simulink model "proc_control_lite"  (R2024b)
settings: Solver=FixedStepAuto  StartTime=0.0  StopTime=inf  RelTol=1e-3
InitFcn:
  | InitProcControl;
StartFcn:
  | LoadParams;
model workspace (MAT data in the model file):
  SL_ROS_VariableLengthArrays_MaxSizes : object (value not decoded)
values from neighbouring files (symbols this model uses):
  A = T200Spec16V{:,3}    [InitProcControl.m]
  N = T200Spec16V{:,6}    [InitProcControl.m]
  PWM = T200Spec16V{:,1}    [InitProcControl.m]
undefined symbols (not defined in the file or in its folder): config, current_gains, DiscIntNeverNeededParam, is_mpc_alive, is_trajectory_done, motor1, motor2, motor3, motor4, motor5, motor6, motor7, motor8, MPC, mpc_mode, mpc_status, orientation, physics, pose, position, simulation, simulink, target_reached, thrusters_status, thrusters_status_SL_Info, twist
libraries: ros2lib x64, dspstat3 x24, aerolibutil x15, dspfdesign x7, simulink x5, mpclib x3, matrix_library x3, robotcorelib x2, sharedtransform x1, sharedTrackingLibrary x1
(part 2 of 3)

== system proc_control_lite/Subsystem Trajectory/ProcPlanner Trajectory ==
  isNew : Inport
  trajMsg : Inport  Port=2
  output : Inport  Port=3
  reset : Inport  Port=4
  rosParam : Inport  Port=5
  Action Port : ActionPort  ActionPortLabel=case [ 10 ]:
  Bus Creator : BusCreator  Inputs=4
  Bus Selector : BusSelector  OutputSignals=WorldPosition,qS2W,Body Velocity,Angular Rate  OutputAsBus=on
  Detect Rise Positive : simulink/Logic and Bit Operations/Detect Rise Positive  vinit=0  OutDataTypeStr=boolean
  MATLAB System : MATLABSystem  System=ProcPlannerManager  mpcConst=MPC  SimulateUsing=Code generation
      mask Type: ProcPlannerManager
      mask Display:
      | disp('ProcPlannerManager');
      | port_label('input',1,'isNew');
      | port_label('input',2,'trajMsg');
      | port_label('input',3,'reset');
      | port_label('input',4,'mesuredPose');
      | port_label('input',5,'mpcParams');
      | port_label('output',1,'currentPose');
      | port_label('output',2,'isReached');
      | port_label('output',3,'isTrajDone');
      | port_label('output',4,'initWpt');
  Refrence : Outport
  wires:
  isNew/1 -> Detect Rise Positive/1
  Detect Rise Positive/1 -> MATLAB System/1
  trajMsg/1 -> MATLAB System/2
  reset/1 -> MATLAB System/3
  output/1 -> Bus Selector/1
  Bus Selector/1 -> MATLAB System/4
  rosParam/1 -> MATLAB System/5
  MATLAB System/4 -> Bus Creator/4  "target"
  MATLAB System/3 -> Bus Creator/3  "isTrajDone"
  MATLAB System/2 -> Bus Creator/2  "isReached"
  MATLAB System/1 -> Bus Creator/1  "Reference"
  Bus Creator/1 -> Refrence/1

== system proc_control_lite/Subsystem Trajectory/Send Current Target ==
  pose : Inport
  Blank Message : ros2lib/Blank Message  messageClass=Message  entityType=geometry_msgs/Pose  messageType=geometry_msgs/Pose  SampleTime=inf
  Bus Assignment : BusAssignment  AssignedSignals=position.x,position.y,position.z,orientation.w,orientation.x,orientation.y,orientation.z
  Demux : Demux  Outputs=7
  Publish : ros2lib/Publish  topicSource=Specify your own  topic=/proc_control/current_target  messageType=geometry_msgs/Pose  QOSHistory=Keep last  QOSDepth=1  QOSReliability=Reliable  QOSDurability=Volatile  QOSDeadline=Inf  QOSLifespan=5  QOSLiveliness=Automatic  QOSLeaseDuration=5  QOSAvoidROSNamespaceConventions=off
  Zero-Order Hold : ZeroOrderHold
  wires:
  Blank Message/1 -> Bus Assignment/1
  pose/1 -> Demux/1
  Demux/1 -> Bus Assignment/2
  Demux/2 -> Bus Assignment/3
  Demux/3 -> Bus Assignment/4
  Demux/4 -> Bus Assignment/5
  Demux/5 -> Bus Assignment/6
  Demux/6 -> Bus Assignment/7
  Demux/7 -> Bus Assignment/8
  Bus Assignment/1 -> Zero-Order Hold/1
  Zero-Order Hold/1 -> Publish/1

== system proc_control_lite/Subsystem Trajectory/SpaceNav ==
  y : Inport
  Action Port : ActionPort  ActionPortLabel=case [ 19 20 21 ]:
  Bus Creator : BusCreator  Inputs=4
  Constant : Constant  Value=[0 0 0 1 0 0 0]
  Constant1 : Constant  Value=MPC.p
  Constant2 : Constant  Value=false  VectorParams1D=off
  Constant3 : Constant  Value=false  VectorParams1D=off
  MATLAB Function : MATLAB Function  TreatAsAtomicUnit=on
  Mux : Mux  Inputs=2
  Selector : Selector  InputPortWidth=13  IndexOptions=Index vector (dialog)  Indices=[1:7]  OutputSizes=1
  Transpose : Math  Operator=transpose  OutputSignalType=real
  Out1 : Outport
  wires:
  Constant/1 -> Mux/1
  y/1 -> Mux/2
  Mux/1 -> Transpose/1
  Transpose/1 -> Selector/1, MATLAB Function/1(matrix)
  Constant1/1 -> MATLAB Function/2(p)
  MATLAB Function/1(y) -> Bus Creator/1  "Reference"
  Selector/1 -> Bus Creator/4  "target"
  Constant3/1 -> Bus Creator/3  "isTrajDone"
  Constant2/1 -> Bus Creator/2  "isReached"
  Bus Creator/1 -> Out1/1

== system proc_control_lite/Subsystem Trajectory/Subsystem ==
  Bus Selector : BusSelector  OutputSignals=linear.x,linear.y,linear.z  OutputAsBus=on
  Bus Selector1 : BusSelector  OutputSignals=angular.x,angular.y,angular.z  OutputAsBus=on
  Bus to Vector : BusToVector
  Bus to Vector1 : BusToVector
  Gain : Gain  Gain=-1
  Mux : Mux  Inputs=2
  Scope : Scope
  Subscribe : ros2lib/Subscribe  topicSource=Specify your own  topic=/spacenav/twist  messageType=geometry_msgs/Twist  sampleTime=1/25  QOSHistory=Keep last  QOSDepth=1  QOSReliability=Reliable  QOSDurability=Volatile  QOSDeadline=Inf  QOSLifespan=5  QOSLiveliness=Automatic  QOSLeaseDuration=5  QOSAvoidROSNamespaceConventions=off
  Terminator : Terminator
  y : Outport
  wires:
  Subscribe/1 -> Terminator/1
  Subscribe/2 -> Bus Selector1/1, Bus Selector/1
  Bus Selector/1 -> Bus to Vector/1
  Bus Selector1/1 -> Bus to Vector1/1
  Bus to Vector1/1 -> Gain/1
  Bus to Vector/1 -> Mux/1
  Gain/1 -> Mux/2
  Mux/1 -> Scope/1, y/1

== system proc_control_lite/Subsystem Trajectory/Subsystem1 ==
  Subscribe : ros2lib/Subscribe  topicSource=Specify your own  topic=/proc_planner/send_trajectory_list  messageType=trajectory_msgs/MultiDOFJointTrajectoryPoint  sampleTime=1  QOSHistory=Keep last  QOSDepth=1  QOSReliability=Reliable  QOSDurability=Volatile  QOSDeadline=Inf  QOSLifespan=inf  QOSLiveliness=Automatic  QOSLeaseDuration=Inf  QOSAvoidROSNamespaceConventions=off
  isNew : Outport
  trajMsg : Outport  Port=2
  wires:
  Subscribe/1 -> isNew/1
  Subscribe/2 -> trajMsg/1

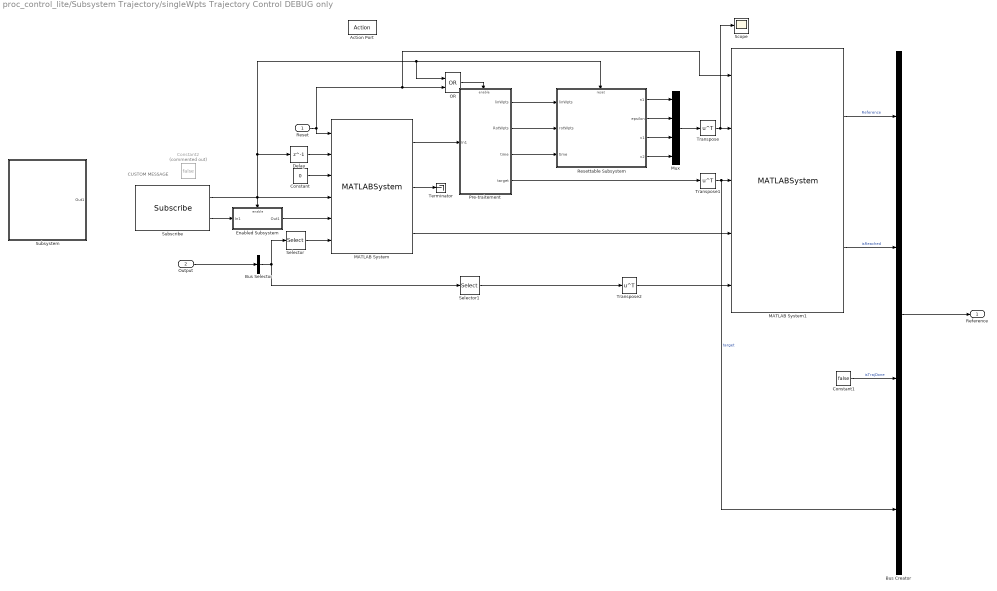
== system proc_control_lite/Subsystem Trajectory/singleWpts Trajectory Control DEBUG only ==
  note: CUSTOM MESSAGE
  Reset : Inport
  Output : Inport  Port=2
  Action Port : ActionPort  InitializeStates=reset  ActionPortLabel=case [ 11 30 31 40 41 ]:
  Bus Creator : BusCreator  Inputs=4
  Bus Selector : BusSelector  OutputSignals=WorldPosition,qS2W,Body Velocity,Angular Rate  OutputAsBus=on
  Constant : Constant  Value=0
  Constant1 : Constant  Value=false
  Constant2 : Constant  Commented=on  Value=false
  Delay : Delay  DelayLength=1
  Enabled Subsystem : Subsystem  TreatAsAtomicUnit=on
  MATLAB System : MATLABSystem  System=AddPose  buffSize=2  elementSize=9  SimulateUsing=Code generation
      mask Type: AddPose
      mask Display:
      | disp('AddPose');
      | port_label('input',1,'reset');
      | port_label('input',2,'compute');
      | port_label('input',3,'clearBuffer');
      | port_label('input',4,'isNew');
      | port_label('input',5,'waypoint');
      | port_label('input',6,'xk');
      | port_label('output',1,'waypoints');
      | port_label('output',2,'count');
      | port_label('output',3,'initCond');
  MATLAB System1 : MATLABSystem  System=TrajectoryManager  SampleTime=MPC.Ts  OffsetTime=0  prediction=MPC.p  bufferSize=6001  linearConvergence=.25  quaternionConvergence=.22  TargetThreshold=2  SimulateUsing=Code generation
      mask Type: TrajectoryManager
      mask Display:
      | disp('TrajectoryManager');
      | port_label('input',1,'reset');
      | port_label('input',2,'poses');
      | port_label('input',3,'target');
      | port_label('input',4,'x0');
      | port_label('input',5,'mesuredPose');
      | port_label('output',1,'currentPose');
      | port_label('output',2,'isReached');
  Mux : Mux
  OR : Logic  Operator=OR  IconShape=distinctive  AllPortsSameDT=off  OutDataTypeStr=boolean
  Pre-traitement : Subsystem  TreatAsAtomicUnit=on
  Resettable Subsystem : Subsystem  TreatAsAtomicUnit=on
  Scope : Scope
  Selector : Selector  InputPortWidth=13  IndexOptions=Index vector (dialog)  Indices=[1:7]  OutputSizes=1
  Selector1 : Selector  InputPortWidth=13  IndexOptions=Index vector (dialog)  Indices=[1:13]  OutputSizes=1
  Subscribe : ros2lib/Subscribe  topicSource=Specify your own  topic=/proc_control/add_pose  messageType=sonia_common_ros2/Pose  sampleTime=-1  QOSHistory=Keep last  QOSDepth=1  QOSReliability=Reliable  QOSDurability=Volatile  QOSDeadline=Inf  QOSLifespan=inf  QOSLiveliness=Automatic  QOSLeaseDuration=inf  QOSAvoidROSNamespaceConventions=off
  Subsystem : Subsystem
  Terminator : Terminator
  Transpose : Math  Operator=transpose
  Transpose1 : Math  Operator=transpose
  Transpose2 : Math  Operator=transpose
  Reference : Outport
  wires:
  Reset/1 -> MATLAB System1/1, OR/2, MATLAB System/1
  Subscribe/1 -> Resettable Subsystem/Reset, OR/1, Delay/1, Enabled Subsystem/Enable, MATLAB System/4
  Enabled Subsystem/1(Out1) -> MATLAB System/5
  Constant/1 -> MATLAB System/3
  Delay/1 -> MATLAB System/2
  MATLAB System/2 -> Terminator/1
  Output/1 -> Bus Selector/1
  Bus Selector/1 -> Selector/1, Selector1/1
  Selector/1 -> MATLAB System/6
  MATLAB System/1 -> Pre-traitement/1(In1)
  OR/1 -> Pre-traitement/Enable
  Pre-traitement/1(linWpts) -> Resettable Subsystem/1(linWpts)
  Pre-traitement/2(RotWpts) -> Resettable Subsystem/2(rotWpts)
  Pre-traitement/3(time) -> Resettable Subsystem/3(time)
  Resettable Subsystem/1(n1) -> Mux/1
  Resettable Subsystem/2(epsilon) -> Mux/2
  Resettable Subsystem/3(v1) -> Mux/3
  Resettable Subsystem/4(v2) -> Mux/4
  Mux/1 -> Transpose/1
  Transpose/1 -> Scope/1, MATLAB System1/2
  Pre-traitement/4(target) -> Transpose1/1
  Transpose1/1 -> Bus Creator/4, MATLAB System1/3  "target"
  MATLAB System/3 -> MATLAB System1/4
  Transpose2/1 -> MATLAB System1/5
  Selector1/1 -> Transpose2/1
  MATLAB System1/1 -> Bus Creator/1  "Reference"
  MATLAB System1/2 -> Bus Creator/2  "isReached"
  Constant1/1 -> Bus Creator/3  "isTrajDone"
  Bus Creator/1 -> Reference/1
  Subscribe/2 -> Enabled Subsystem/1(In1)

== system proc_control_lite/Enabled Subsystem/Send auv states/bus2mux ==
  Input : Inport
  Bus Selector : BusSelector  OutputSignals=WorldPosition,qS2W,Body Velocity,Angular Rate
  Mux : Mux
  states : Outport
  wires:
  Bus Selector/1 -> Mux/1  "<WorldPosition>"
  Input/1 -> Bus Selector/1
  Bus Selector/2 -> Mux/2  "<qS2W>"
  Mux/1 -> states/1
  Bus Selector/3 -> Mux/3  "<Body Velocity>"
  Bus Selector/4 -> Mux/4  "<Angular Rate>"

== system proc_control_lite/Ros Command/Get_ROS_param/MPC Parameters ==
  Bus Creator : BusCreator  Inputs=2  OutDataTypeStr=Bus: mpcParams
  MPC Gains : Subsystem
  targetReached Params : Subsystem
  mpcParams : Outport
  wires:
  MPC Gains/1(gains) -> Bus Creator/1
  targetReached Params/1(targetReached) -> Bus Creator/2
  Bus Creator/1 -> mpcParams/1  "mpcParams"

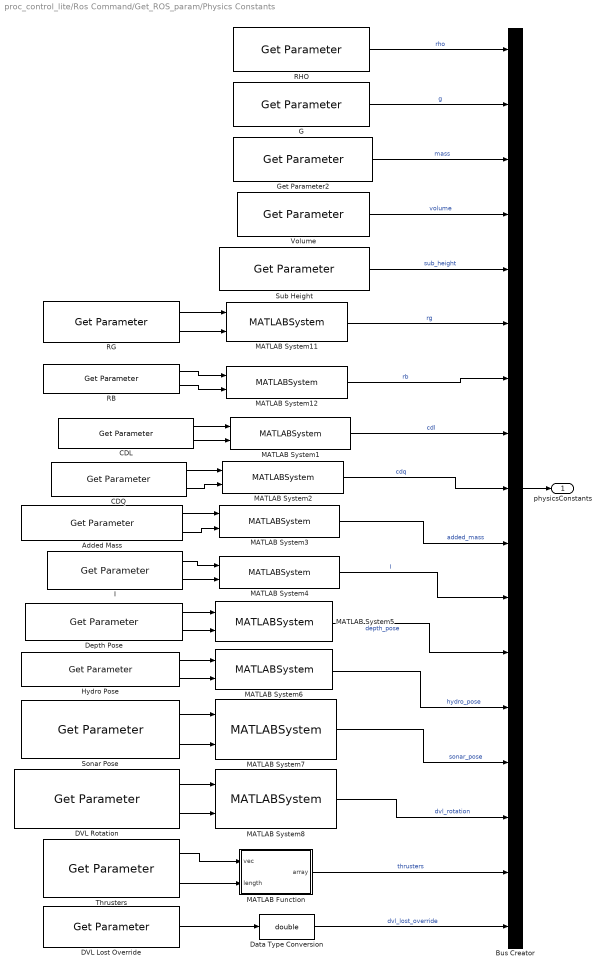
== system proc_control_lite/Ros Command/Get_ROS_param/Physics Constants ==
  Added Mass : ros2lib/Get Parameter  ParameterName=proc_control.physics.added_mass  ParameterType=double[]  ParameterMaxArrayLength=64  ParameterInitialValue=int8([0,0,0,0,0,0])  SampleTime=-1  ModelName=proc_control_lite  BlockId=ParamGet_proc_control_lite_180
  Bus Creator : BusCreator  Inputs=17  OutDataTypeStr=Bus: physicsConstants  NonVirtualBus=on
  CDL : ros2lib/Get Parameter  ParameterName=proc_control.physics.cdl  ParameterType=double[]  ParameterMaxArrayLength=64  ParameterInitialValue=int8([0,0,0,0,0,0])  SampleTime=-1  ModelName=proc_control_lite  BlockId=ParamGet_proc_control_lite_175
  CDQ : ros2lib/Get Parameter  ParameterName=proc_control.physics.cdq  ParameterType=double[]  ParameterMaxArrayLength=64  ParameterInitialValue=int8([0,0,0,0,0,0])  SampleTime=-1  ModelName=proc_control_lite  BlockId=ParamGet_proc_control_lite_177
  DVL Lost Override : ros2lib/Get Parameter  ParameterName=proc_control.physics.dvl_lost_override  ParameterType=boolean  ParameterMaxArrayLength=16  ParameterInitialValue=true  SampleTime=-1  ModelName=proc_control_lite  BlockId=ParamGet_proc_control_lite_196
  DVL Rotation : ros2lib/Get Parameter  ParameterName=proc_control.physics.dvl_rotation  ParameterType=double[]  ParameterMaxArrayLength=64  ParameterInitialValue=int8([0,0,0])  SampleTime=-1  ModelName=proc_control_lite  BlockId=ParamGet_proc_control_lite_192
  Data Type Conversion : DataTypeConversion  OutDataTypeStr=double  SaturateOnIntegerOverflow=off  RndMeth=Floor
  Depth Pose : ros2lib/Get Parameter  ParameterName=proc_control.physics.depth_pose  ParameterType=double[]  ParameterMaxArrayLength=64  ParameterInitialValue=int8([0,0,0])  SampleTime=-1  ModelName=proc_control_lite  BlockId=ParamGet_proc_control_lite_184
  G : ros2lib/Get Parameter  ParameterName=proc_control.physics.g  ParameterType=double  ParameterMaxArrayLength=16  ParameterInitialValue=physics.g  SampleTime=-1  ModelName=proc_control_lite  BlockId=ParamGet_proc_control_lite_167
  Get Parameter2 : ros2lib/Get Parameter  ParameterName=proc_control.physics.mass  ParameterType=double  ParameterMaxArrayLength=16  ParameterInitialValue=physics.mass  SampleTime=-1  ModelName=proc_control_lite  BlockId=ParamGet_proc_control_lite_168
  Hydro Pose : ros2lib/Get Parameter  ParameterName=proc_control.physics.hydro_pose  ParameterType=double[]  ParameterMaxArrayLength=64  ParameterInitialValue=int8([0,0,0])  SampleTime=-1  ModelName=proc_control_lite  BlockId=ParamGet_proc_control_lite_186
  I : ros2lib/Get Parameter  ParameterName=proc_control.physics.I  ParameterType=double[]  ParameterMaxArrayLength=128  ParameterInitialValue=int8([0,0,0,0,0,0,0,0,0])  SampleTime=-1  ModelName=proc_control_lite  BlockId=ParamGet_proc_control_lite_182
  MATLAB Function : MATLAB Function  TreatAsAtomicUnit=on
  MATLAB System1 : MATLABSystem  System=Vector2DoubleArray  arraySize=[1, 6]  constantName='Linear drag constant'  SimulateUsing=Code generation
      mask Type: Vector2DoubleArray
      mask Display:
      | disp('Vector2DoubleArray');
      | port_label('input',1,'vector');
      | port_label('input',2,'length');
      | port_label('output',1,'array');
  MATLAB System11 : MATLABSystem  System=Vector2DoubleArray  arraySize=[1 3]  constantName='Center of Mass'  SimulateUsing=Code generation
      mask Type: Vector2DoubleArray
      mask Display:
      | disp('Vector2DoubleArray');
      | port_label('input',1,'vector');
      | port_label('input',2,'length');
      | port_label('output',1,'array');
  MATLAB System12 : MATLABSystem  System=Vector2DoubleArray  arraySize=[1, 3]  constantName='Center of Buoyancy'  SimulateUsing=Code generation
      mask Type: Vector2DoubleArray
      mask Display:
      | disp('Vector2DoubleArray');
      | port_label('input',1,'vector');
      | port_label('input',2,'length');
      | port_label('output',1,'array');
  MATLAB System2 : MATLABSystem  System=Vector2DoubleArray  arraySize=[1, 6]  constantName='Quadratic drag constant'  SimulateUsing=Code generation
      mask Type: Vector2DoubleArray
      mask Display:
      | disp('Vector2DoubleArray');
      | port_label('input',1,'vector');
      | port_label('input',2,'length');
      | port_label('output',1,'array');
  MATLAB System3 : MATLABSystem  System=Vector2DoubleArray  arraySize=[1, 6]  constantName='Added Mass'  SimulateUsing=Code generation
      mask Type: Vector2DoubleArray
      mask Display:
      | disp('Vector2DoubleArray');
      | port_label('input',1,'vector');
      | port_label('input',2,'length');
      | port_label('output',1,'array');
  MATLAB System4 : MATLABSystem  System=Vector2DoubleArray  arraySize=[1,9]  constantName='Inertia Tensor'  SimulateUsing=Code generation
      mask Type: Vector2DoubleArray
      mask Display:
      | disp('Vector2DoubleArray');
      | port_label('input',1,'vector');
      | port_label('input',2,'length');
      | port_label('output',1,'array');
  MATLAB System5 : MATLABSystem  System=Vector2DoubleArray  arraySize=[1 3]  constantName='Depth Pose'  SimulateUsing=Code generation
      mask Type: Vector2DoubleArray
      mask Display:
      | disp('Vector2DoubleArray');
      | port_label('input',1,'vector');
      | port_label('input',2,'length');
      | port_label('output',1,'array');
  MATLAB System6 : MATLABSystem  System=Vector2DoubleArray  arraySize=[1, 3]  constantName='Hydro Pose'  SimulateUsing=Code generation
      mask Type: Vector2DoubleArray
      mask Display:
      | disp('Vector2DoubleArray');
      | port_label('input',1,'vector');
      | port_label('input',2,'length');
      | port_label('output',1,'array');
  MATLAB System7 : MATLABSystem  System=Vector2DoubleArray  arraySize=[1, 3]  constantName='Sonar Pose'  SimulateUsing=Code generation
      mask Type: Vector2DoubleArray
      mask Display:
      | disp('Vector2DoubleArray');
      | port_label('input',1,'vector');
      | port_label('input',2,'length');
      | port_label('output',1,'array');
  MATLAB System8 : MATLABSystem  System=Vector2DoubleArray  arraySize=[1, 3]  constantName='DVL Rotation'  SimulateUsing=Code generation
      mask Type: Vector2DoubleArray
      mask Display:
      | disp('Vector2DoubleArray');
      | port_label('input',1,'vector');
      | port_label('input',2,'length');
      | port_label('output',1,'array');
  RB : ros2lib/Get Parameter  ParameterName=proc_control.physics.rb  ParameterType=double[]  ParameterMaxArrayLength=64  ParameterInitialValue=int8([0,0,0])  SampleTime=-1  ModelName=proc_control_lite  BlockId=ParamGet_proc_control_lite_173
  RG : ros2lib/Get Parameter  ParameterName=proc_control.physics.rg  ParameterType=double[]  ParameterMaxArrayLength=64  ParameterInitialValue=double([0,0,0])  SampleTime=-1  ModelName=proc_control_lite  BlockId=ParamGet_proc_control_lite_171
  RHO : ros2lib/Get Parameter  ParameterName=proc_control.physics.rho  ParameterType=double  ParameterMaxArrayLength=16  ParameterInitialValue=physics.rho  SampleTime=-1  ModelName=proc_control_lite  BlockId=ParamGet_proc_control_lite_166
  Sonar Pose : ros2lib/Get Parameter  ParameterName=proc_control.physics.sonar_pose  ParameterType=double[]  ParameterMaxArrayLength=64  ParameterInitialValue=int8([0,0,0])  SampleTime=-1  ModelName=proc_control_lite  BlockId=ParamGet_proc_control_lite_190
  Sub Height : ros2lib/Get Parameter  ParameterName=proc_control.physics.sub_height  ParameterType=double  ParameterMaxArrayLength=16  ParameterInitialValue=physics.height  SampleTime=-1  ModelName=proc_control_lite  BlockId=ParamGet_proc_control_lite_170
  Thrusters : ros2lib/Get Parameter  ParameterName=proc_control.physics.thrusters  ParameterType=double[]  ParameterMaxArrayLength=400  ParameterInitialValue=int8(zeros(1,48))  SampleTime=-1  ModelName=proc_control_lite  BlockId=ParamGet_proc_control_lite_194
  Volume : ros2lib/Get Parameter  ParameterName=proc_control.physics.volume  ParameterType=double  ParameterMaxArrayLength=16  ParameterInitialValue=physics.volume  SampleTime=-1  ModelName=proc_control_lite  BlockId=ParamGet_proc_control_lite_169
  physicsConstants : Outport
  wires:
  MATLAB System6/1 -> Bus Creator/13  "hydro_pose"
  CDL/2 -> MATLAB System1/2
  MATLAB System2/1 -> Bus Creator/9  "cdq"
  Thrusters/1 -> MATLAB Function/1(vec)
  RG/2 -> MATLAB System11/2
  CDQ/2 -> MATLAB System2/2
  Depth Pose/1 -> MATLAB System5/1
  MATLAB System8/1 -> Bus Creator/15  "dvl_rotation"
  CDL/1 -> MATLAB System1/1
  CDQ/1 -> MATLAB System2/1
  Added Mass/1 -> MATLAB System3/1
  Added Mass/2 -> MATLAB System3/2
  I/1 -> MATLAB System4/1
  I/2 -> MATLAB System4/2
  Depth Pose/2 -> MATLAB System5/2
  Hydro Pose/1 -> MATLAB System6/1
  Hydro Pose/2 -> MATLAB System6/2
  Sonar Pose/1 -> MATLAB System7/1
  Sonar Pose/2 -> MATLAB System7/2
  DVL Rotation/1 -> MATLAB System8/1
  DVL Rotation/2 -> MATLAB System8/2
  Thrusters/2 -> MATLAB Function/2(length)
  DVL Lost Override/1 -> Data Type Conversion/1
  RHO/1 -> Bus Creator/1  "rho"
  Sub Height/1 -> Bus Creator/5  "sub_height"
  G/1 -> Bus Creator/2  "g"
  Volume/1 -> Bus Creator/4  "volume"
  MATLAB System12/1 -> Bus Creator/7  "rb"
  MATLAB System1/1 -> Bus Creator/8  "cdl"
  MATLAB System3/1 -> Bus Creator/10  "added_mass"
  MATLAB System4/1 -> Bus Creator/11  "I"
  MATLAB System5/1 -> Bus Creator/12  "depth_pose"
  MATLAB System7/1 -> Bus Creator/14  "sonar_pose"
  MATLAB Function/1(array) -> Bus Creator/16  "thrusters"
  Data Type Conversion/1 -> Bus Creator/17  "dvl_lost_override"
  Bus Creator/1 -> physicsConstants/1
  Get Parameter2/1 -> Bus Creator/3  "mass"
  RG/1 -> MATLAB System11/1
  MATLAB System11/1 -> Bus Creator/6  "rg"
  RB/1 -> MATLAB System12/1
  RB/2 -> MATLAB System12/2

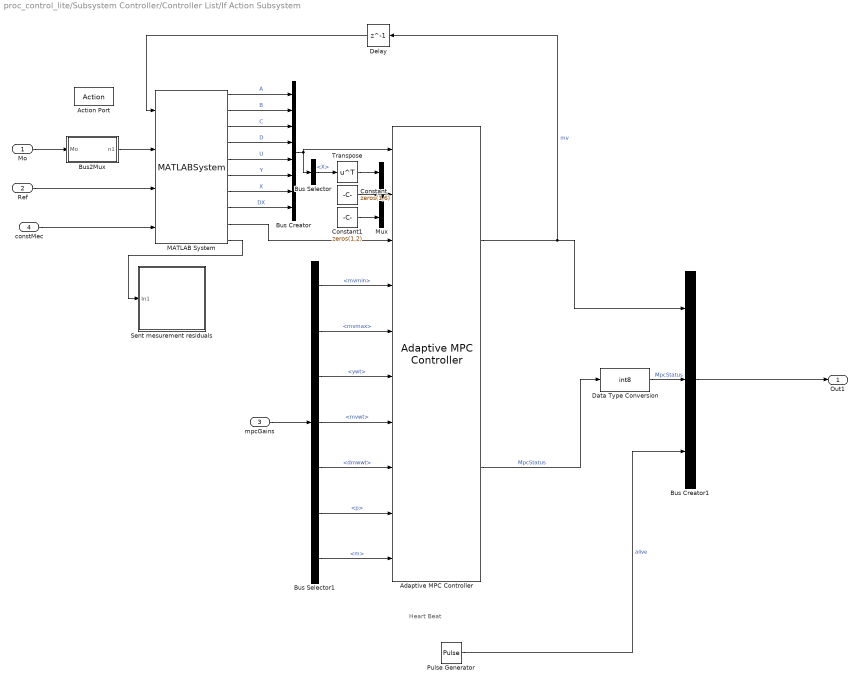
== system proc_control_lite/Subsystem Controller/Controller List/If Action Subsystem ==
  note: Heart Beat
  Mo : Inport
  Ref : Inport  Port=2
  mpcGains : Inport  Port=3
  constMec : Inport  Port=4
  Action Port : ActionPort  InitializeStates=reset  PropagateVarSize=During execution  ActionPortLabel=case [ 10 11 19 31 ]:
  Adaptive MPC Controller : mpclib/Adaptive MPC Controller  SCDEnableBlockLinearizationSpecification=on  mpcobj=Qmpcobj  enable_value=0  updateMPCinCallerWorkspace=on  md_inport=off  mv_inport=off  uref_inport=off  return_cost=off  return_mvseq=off  return_qpstatus=on  return_xseq=off  return_state=off  return_ovseq=off  state_inport=on  isltv_plant=off  umin_inport=on  umax_inport=on  ymin_inport=off  ymax_inport=off  cc_inport=off  ywt_inport=on  uwt_inport=on  duwt_inport=on  rhoeps_inport=off  pm_inport=on  MaximumP=10  HorizonChoice=VariableHorizon  BlockDataType=double  SampleTimeInherited=off  switch_inport=off
  Bus Creator : BusCreator  Inputs=8
  Bus Creator1 : BusCreator  Inputs=3
  Bus Selector : BusSelector  OutputSignals=X
  Bus Selector1 : BusSelector  OutputSignals=mvmin,mvmax,ywt,mvwt,dmwwt,p,m
  Bus2Mux : Subsystem
  Constant : Constant  Value=zeros(1,6)
  Constant1 : Constant  Value=zeros(1,2)
  Data Type Conversion : DataTypeConversion  OutDataTypeStr=int8  SaturateOnIntegerOverflow=off  RndMeth=Floor
  Delay : Delay  DelayLength=1  InitialCondition=zeros(MPC.nu,1)  SampleTime=MPC.Ts
  MATLAB System : MATLABSystem  System=TrimPlant  MPC=MPC  useDynamicsConst=on  SimulateUsing=Code generation
      mask Type: TrimPlant
      mask Display:
      | disp('TrimPlant');
      | port_label('input',1,'u');
      | port_label('input',2,'y');
      | port_label('input',3,'ref');
      | port_label('input',4,'constMec');
      | port_label('output',1,'A');
      | port_label('output',2,'B');
      | port_label('output',3,'C');
      | port_label('output',4,'D');
      | port_label('output',5,'U');
      | port_label('output',6,'Y');
      | port_label('output',7,'X');
      | port_label('output',8,'DX');
      | port_label('output',9,'ref');
      | port_label('output',10,'Z');
  Mux : Mux  Inputs=3
  Pulse Generator : DiscretePulseGenerator  SampleTime=MPC.Ts
  Sent mesurement residuals : Subsystem
  Transpose : Math  Operator=transpose
  Out1 : Outport
  wires:
  Mo/1 -> Bus2Mux/1(Mo)
  Bus2Mux/1(n1) -> MATLAB System/2
  Ref/1 -> MATLAB System/3
  constMec/1 -> MATLAB System/4
  MATLAB System/1 -> Bus Creator/1  "A"
  MATLAB System/2 -> Bus Creator/2  "B"
  MATLAB System/3 -> Bus Creator/3  "C"
  MATLAB System/4 -> Bus Creator/4  "D"
  MATLAB System/5 -> Bus Creator/5  "U"
  MATLAB System/6 -> Bus Creator/6  "Y"
  MATLAB System/7 -> Bus Creator/7  "X"
  MATLAB System/8 -> Bus Creator/8  "DX"
  Bus Creator/1 -> Bus Selector/1, Adaptive MPC Controller/1
  Constant/1 -> Mux/2
  Constant1/1 -> Mux/3
  Mux/1 -> Adaptive MPC Controller/2
  Bus Selector/1 -> Transpose/1  "<X>"
  Transpose/1 -> Mux/1
  MATLAB System/9 -> Adaptive MPC Controller/3
  mpcGains/1 -> Bus Selector1/1
  Bus Selector1/1 -> Adaptive MPC Controller/4  "<mvmin>"
  Bus Selector1/2 -> Adaptive MPC Controller/5  "<mvmax>"
  Bus Selector1/3 -> Adaptive MPC Controller/6  "<ywt>"
  Bus Selector1/4 -> Adaptive MPC Controller/7  "<mvwt>"
  Bus Selector1/5 -> Adaptive MPC Controller/8  "<dmwwt>"
  Bus Selector1/6 -> Adaptive MPC Controller/9  "<p>"
  Bus Selector1/7 -> Adaptive MPC Controller/10  "<m>"
  MATLAB System/10 -> Sent mesurement residuals/1(In1)
  Adaptive MPC Controller/1 -> Delay/1, Bus Creator1/1  "mv"
  Adaptive MPC Controller/2 -> Data Type Conversion/1  "MpcStatus"
  Pulse Generator/1 -> Bus Creator1/3  "alive"
  Delay/1 -> MATLAB System/1
  Bus Creator1/1 -> Out1/1
  Data Type Conversion/1 -> Bus Creator1/2  "MpcStatus"

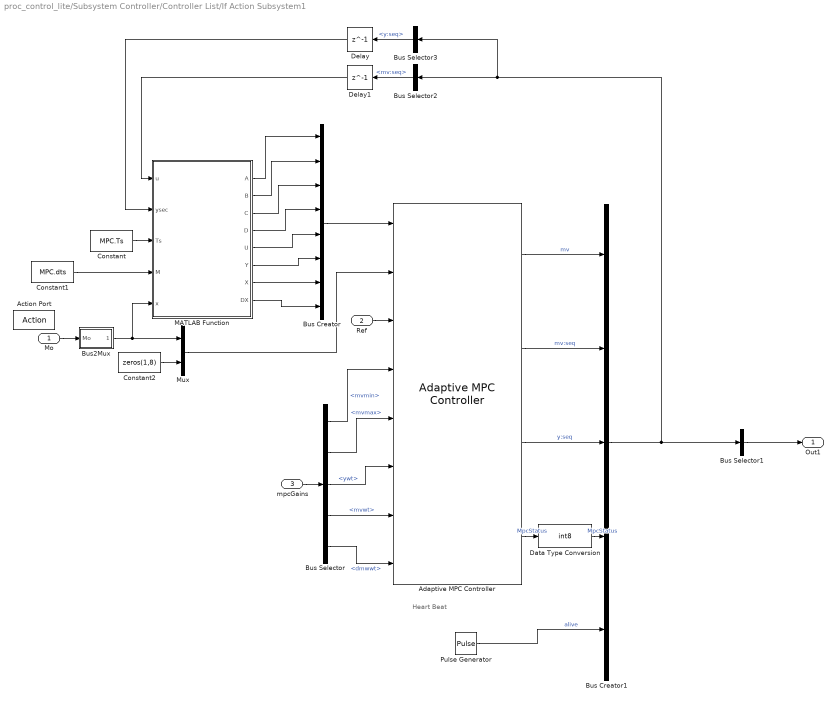
== system proc_control_lite/Subsystem Controller/Controller List/If Action Subsystem1 ==
  note: Heart Beat
  Mo : Inport
  Ref : Inport  Port=2
  mpcGains : Inport  Port=3
  Action Port : ActionPort  InitializeStates=reset  PropagateVarSize=During execution  ActionPortLabel=case [ 30 ]:
  Adaptive MPC Controller : mpclib/Adaptive MPC Controller  SCDEnableBlockLinearizationSpecification=on  mpcobj=Qmpcobj  enable_value=0  updateMPCinCallerWorkspace=on  md_inport=off  mv_inport=off  uref_inport=off  return_cost=off  return_mvseq=on  return_qpstatus=on  return_xseq=off  return_state=off  return_ovseq=on  state_inport=on  isltv_plant=on  umin_inport=on  umax_inport=on  ymin_inport=off  ymax_inport=off  cc_inport=off  ywt_inport=on  uwt_inport=on  duwt_inport=on  rhoeps_inport=off  pm_inport=off  MaximumP=10  HorizonChoice=FixedHorizon  BlockDataType=double  SampleTimeInherited=off  switch_inport=off
  Bus Creator : BusCreator  Inputs=8
  Bus Creator1 : BusCreator  Inputs=5
  Bus Selector : BusSelector  OutputSignals=mvmin,mvmax,ywt,mvwt,dmwwt
  Bus Selector1 : BusSelector  OutputSignals=mv,MpcStatus,alive  OutputAsBus=on
  Bus Selector2 : BusSelector  OutputSignals=mv:seq
  Bus Selector3 : BusSelector  OutputSignals=y:seq
  Bus2Mux : Subsystem
  Constant : Constant  Value=MPC.Ts
  Constant1 : Constant  Value=MPC.dts
  Constant2 : Constant  Value=zeros(1,8)
  Data Type Conversion : DataTypeConversion  OutDataTypeStr=int8  SaturateOnIntegerOverflow=off  RndMeth=Floor
  Delay : Delay  DelayLength=1  InitialCondition=repmat(MPC.Xi.',11,1)  SampleTime=MPC.Ts
  Delay1 : Delay  DelayLength=1  InitialCondition=zeros(11,8)  SampleTime=MPC.Ts
  MATLAB Function : MATLAB Function  TreatAsAtomicUnit=on
  Mux : Mux  Inputs=2
  Pulse Generator : DiscretePulseGenerator  SampleTime=MPC.Ts
  Out1 : Outport
  wires:
  MATLAB Function/2(B) -> Bus Creator/2
  Mo/1 -> Bus2Mux/1(Mo)
  Constant/1 -> MATLAB Function/3(Ts)
  Constant1/1 -> MATLAB Function/4(M)
  Bus Selector/5 -> Adaptive MPC Controller/8  "<dmwwt>"
  MATLAB Function/7(X) -> Bus Creator/7
  Bus2Mux/1(Out1) -> Mux/1, MATLAB Function/5(x)
  Constant2/1 -> Mux/2
  MATLAB Function/3(C) -> Bus Creator/3
  MATLAB Function/1(A) -> Bus Creator/1
  Ref/1 -> Adaptive MPC Controller/3
  Mux/1 -> Adaptive MPC Controller/2
  MATLAB Function/4(D) -> Bus Creator/4
  MATLAB Function/5(U) -> Bus Creator/5
  MATLAB Function/6(Y) -> Bus Creator/6
  MATLAB Function/8(DX) -> Bus Creator/8
  mpcGains/1 -> Bus Selector/1
  Bus Creator/1 -> Adaptive MPC Controller/1
  Bus Selector/2 -> Adaptive MPC Controller/5  "<mvmax>"
  Bus Selector/1 -> Adaptive MPC Controller/4  "<mvmin>"
  Bus Selector/3 -> Adaptive MPC Controller/6  "<ywt>"
  Bus Selector/4 -> Adaptive MPC Controller/7  "<mvwt>"
  Adaptive MPC Controller/1 -> Bus Creator1/1  "mv"
  Adaptive MPC Controller/4 -> Data Type Conversion/1  "MpcStatus"
  Adaptive MPC Controller/3 -> Bus Creator1/3  "y:seq"
  Adaptive MPC Controller/2 -> Bus Creator1/2  "mv:seq"
  Pulse Generator/1 -> Bus Creator1/5  "alive"
  Bus Selector1/1 -> Out1/1
  Bus Creator1/1 -> Bus Selector3/1, Bus Selector2/1, Bus Selector1/1
  Bus Selector3/1 -> Delay/1  "<y:seq>"
  Bus Selector2/1 -> Delay1/1  "<mv:seq>"
  Delay1/1 -> MATLAB Function/1(u)
  Delay/1 -> MATLAB Function/2(ysec)
  Data Type Conversion/1 -> Bus Creator1/4  "MpcStatus"

== system proc_control_lite/Subsystem Controller/Controller List/If Action Subsystem2 ==
  mo : Inport
  ref : Inport  Port=2
  mode : Inport  Port=3
  Action Port : ActionPort  ActionPortLabel=case [ 20 21 ]:
  Bus Creator : BusCreator  Inputs=3
  Constant : Constant  Value=int8(0)
  Constant1 : Constant  Value=0
  Discrete Derivative : simulink/Discrete/Discrete Derivative  gainval=1.0  ICPrevScaledInput=0.0  OutMin=[]  OutMax=[]  OutDataType=fixdt(1, 16)  OutScaling=2^-10  DoSatur=off
  MATLAB System : MATLABSystem  System=OpenLoopController  k=40  binv=binv  mass=physics.mass  volume=physics.volume  height=physics.height  I=physics.I  RG=physics.RG  RB=physics.RB  AddedMass=physics.AddedMass  CDL=physics.CDL  CDQ=physics.CDQ  AF=physics.AF  g=physics.g  rho=physics.rho  SimulateUsing=Code generation
      mask Type: OpenLoopController
      mask Display:
      | disp('OpenLoopController');
      | port_label('input',1,'ref');
      | port_label('input',2,'ref_dot');
      | port_label('input',3,'mo');
      | port_label('input',4,'mode');
      | port_label('output',1,'mv');
  Reshape : Reshape
  Selector : Selector  NumberOfDimensions=2  InputPortWidth=3  IndexOptions=Index vector (dialog),Index vector (dialog)  Indices=1,[8:13]  OutputSizes=1,1
  Out1 : Outport
  wires:
  mode/1 -> MATLAB System/4
  ref/1 -> Selector/1
  Selector/1 -> MATLAB System/1, Discrete Derivative/1
  Discrete Derivative/1 -> MATLAB System/2
  Reshape/1 -> Bus Creator/1  "mv"
  MATLAB System/1 -> Reshape/1
  mo/1 -> MATLAB System/3
  Constant/1 -> Bus Creator/2  "MpcStatus"
  Constant1/1 -> Bus Creator/3  "alive"
  Bus Creator/1 -> Out1/1

== system proc_control_lite/Subsystem Controller/Controller List/If Action Subsystem3 ==
  Action Port : ActionPort  ActionPortLabel=default:
  Bus Creator : BusCreator  Inputs=3
  Constant : Constant  Value=zeros(1,MPC.nu)
  Constant1 : Constant  Value=int8(0)
  Constant2 : Constant  Value=0
  Out1 : Outport
  wires:
  Constant/1 -> Bus Creator/1  "mv"
  Constant1/1 -> Bus Creator/2  "MpcStatus"
  Constant2/1 -> Bus Creator/3  "alive"
  Bus Creator/1 -> Out1/1

== system proc_control_lite/Subsystem Controller/Controller List/Quaternion Non linear MPC (Not for codegen) ==
  note: Heart beat
  Mo : Inport
  Ref : Inport  Port=2
  mpc Gains : Inport  Port=3
  Action Port : ActionPort  InitializeStates=reset  ActionPortLabel=case [ 40 ]:
  Bus Creator : BusCreator  Inputs=3
  Bus Selector : BusSelector  OutputSignals=mvmin,mvmax,ywt,mvwt,dmwwt
  Bus2Mux1 : Subsystem
  Data Type Conversion : DataTypeConversion  OutDataTypeStr=int8  SaturateOnIntegerOverflow=off  RndMeth=Floor
  Delay : Delay  DelayLength=1  InitialCondition=zeros(MPC.nu,1)
  Nonlinear MPC Controller : mpclib/Nonlinear MPC Controller  nlmpcobj=nlobj  UseObjectTs=on  TsControl=0.02  UseMEX=off  md_enabled=off  mvtarget_enabled=off  param_enabled=off  cost_enabled=off  mvseq_enabled=off  stateseq_enabled=off  ovseq_enabled=off  slack_enabled=off  status_enabled=on  ov_min=off  ov_max=off  mv_min=on  mv_max=on  mvrate_min=off  mvrate_max=off  state_min=off  state_max=off  ov_weight=on  mv_weight=on  mvrate_weight=on  ecr_weight=off  nlp_initialize=off
  Pulse Generator : DiscretePulseGenerator  Period=20  PulseWidth=10  SampleTime=MPC.Ts
  Out : Outport
  wires:
  Mo/1 -> Bus2Mux1/1(Mo)
  Bus2Mux1/1(Out1) -> Nonlinear MPC Controller/1
  Ref/1 -> Nonlinear MPC Controller/2
  mpc Gains/1 -> Bus Selector/1
  Bus Selector/1 -> Nonlinear MPC Controller/4  "<mvmin>"
  Bus Selector/2 -> Nonlinear MPC Controller/5  "<mvmax>"
  Bus Selector/3 -> Nonlinear MPC Controller/6  "<ywt>"
  Bus Selector/4 -> Nonlinear MPC Controller/7  "<mvwt>"
  Bus Selector/5 -> Nonlinear MPC Controller/8  "<dmwwt>"
  Nonlinear MPC Controller/1 -> Bus Creator/1, Delay/1  "mv"
  Delay/1 -> Nonlinear MPC Controller/3
  Nonlinear MPC Controller/2 -> Data Type Conversion/1  "MpcStatus"
  Pulse Generator/1 -> Bus Creator/3  "alive"
  Bus Creator/1 -> Out/1
  Data Type Conversion/1 -> Bus Creator/2  "MpcStatus"

== system proc_control_lite/Subsystem Controller/If Action Subsystem/Subsystem ==
  Bus Creator : BusCreator  Inputs=8
  Constant : Constant  Value=zeros(1, 128)
  Constant1 : Constant  Value=zeros(1, 128)
  Constant2 : Constant  Value=zeros(1, 128)
  Constant3 : Constant  Value=MPC.tmax
  Constant4 : Constant  Value=MPC.tmin
  Subsystem : Subsystem
  Subsystem1 : Subsystem
  Subsystem2 : Subsystem
  Out1 : Outport
  wires:
  Constant4/1 -> Bus Creator/8  "min_thrust"
  Constant2/1 -> Bus Creator/5  "mvr"
  Constant3/1 -> Bus Creator/7  "max_thrust"
  Constant/1 -> Bus Creator/1  "ov"
  Subsystem/1(Out1) -> Bus Creator/2  "ov_SL_Info"
  Subsystem2/1(Out1) -> Bus Creator/4  "mv_SL_Info"
  Constant1/1 -> Bus Creator/3  "mv"
  Subsystem1/1(Out1) -> Bus Creator/6  "mvr_SL_Info"
  Bus Creator/1 -> Out1/1

== system proc_control_lite/Subsystem ProcNav/AHRS//Detph Mesurments/Acceleration to velocity ==
  q : Inport
  vec : Inport  Port=2
  Angular Rate : Inport  Port=3
  SensorOn : Inport  Port=4
  Normal mode : Subsystem  VariantControl=SimulationActive==2
  Simulation : Subsystem  VariantControl=SimulationActive==1
  vec_rot : Outport

== system proc_control_lite/Subsystem ProcNav/AHRS//Detph Mesurments/Acceleration to velocity ZED ==
  q : Inport
  vec : Inport  Port=2
  Angular Rate : Inport  Port=3
  SensorOn : Inport  Port=4
  Normal mode : Subsystem  VariantControl=SimulationActive==2
  Subsystem1 : Subsystem  VariantControl=SimulationActive==1
  vec_rot : Outport

== system proc_control_lite/Subsystem ProcNav/DVL Measurements/DVL2Ship ==
  dvl Rotation : Inport
  Constant : Constant  Value=0
  Delay : Delay  DelayLength=1  InitialCondition=1
  Enabled Subsystem : Subsystem  TreatAsAtomicUnit=on
  Quat : Outport
  wires:
  Constant/1 -> Delay/1
  Delay/1 -> Enabled Subsystem/Enable
  dvl Rotation/1 -> Enabled Subsystem/1(dvl Rotation)
  Enabled Subsystem/1(Quat) -> Quat/1

== system proc_control_lite/Subsystem ProcNav/Enabled Subsystem/Subsystem ==
  mecConst : Inport
  In2 : Inport  Port=2
  Bus Selector : BusSelector  OutputSignals=dvl_lost_override
  Bus Selector1 : BusSelector  OutputSignals=enable,Body Velocity
  Constant : Constant  Value=0
  Constant1 : Constant  Value=0
  Constant3 : Constant  Value=config.dvl
  Constant4 : Constant  Value=config.dvl
  Mux1 : Mux  Inputs=3
  Random Number : RandomNumber  Variance=0.0000000001  Seed=1  SampleTime=0.02
  Random Number1 : RandomNumber  Variance=0.0000000001  Seed=525886  SampleTime=0.02
  Random Number2 : RandomNumber  Variance=0.0000000001  Seed=4  SampleTime=0.02
  Switch : Switch  Criteria=u2 > Threshold  SaturateOnIntegerOverflow=off  InputSameDT=off
  Switch1 : Switch  Criteria=u2 > Threshold  SaturateOnIntegerOverflow=off  InputSameDT=off
  Switch2 : Switch  Criteria=u2 > Threshold  SaturateOnIntegerOverflow=off  InputSameDT=off
  Zero-Order Hold : ZeroOrderHold  SampleTime=simulink.procNav.dvl.sampletime
  Out1 : Outport
  y1 : Outport  Port=2
  wires:
  Bus Selector1/1 -> Switch/3  "<enable>"
  In2/1 -> Bus Selector1/1
  Constant/1 -> Switch/1
  Bus Selector1/2 -> Zero-Order Hold/1  "<Body Velocity>"
  Bus Selector/1 -> Switch/2  "<dvl_lost_override>"
  Zero-Order Hold/1 -> Switch2/1
  Switch/1 -> Switch1/1
  mecConst/1 -> Bus Selector/1
  Constant3/1 -> Switch1/2
  Constant1/1 -> Switch1/3
  Switch1/1 -> Out1/1
  Constant4/1 -> Switch2/2
  Mux1/1 -> Switch2/3
  Switch2/1 -> y1/1
  Random Number2/1 -> Mux1/3
  Random Number1/1 -> Mux1/1
  Random Number/1 -> Mux1/2

== system proc_control_lite/Subsystem Trajectory/singleWpts Trajectory Control DEBUG only/Enabled Subsystem ==
  In1 : Inport
  Enable : EnablePort
  Bus Selector : BusSelector  OutputSignals=frame,speed  OutputAsBus=on
  Bus Selector1 : BusSelector  OutputSignals=position.x,position.y,position.z,orientation.z,orientation.y,orientation.x  OutputAsBus=on
  Bus Selector2 : BusSelector  OutputSignals=fine  OutputAsBus=on
  Data Type Conversion : DataTypeConversion  OutDataTypeStr=double  SaturateOnIntegerOverflow=off  RndMeth=Floor  LockScale=on
  Data Type Conversion1 : DataTypeConversion  OutDataTypeStr=double  SaturateOnIntegerOverflow=off  RndMeth=Floor  LockScale=on
  Data Type Conversion2 : DataTypeConversion  OutDataTypeStr=double  SaturateOnIntegerOverflow=off  RndMeth=Floor  LockScale=on
  Mux : Mux  Inputs=3
  Out1 : Outport
  wires:
  In1/1 -> Bus Selector2/1, Bus Selector1/1, Bus Selector/1
  Bus Selector1/1 -> Data Type Conversion/1
  Bus Selector2/1 -> Data Type Conversion2/1
  Bus Selector/1 -> Data Type Conversion1/1
  Mux/1 -> Out1/1
  Data Type Conversion/1 -> Mux/1
  Data Type Conversion1/1 -> Mux/2
  Data Type Conversion2/1 -> Mux/3

== system proc_control_lite/Subsystem Trajectory/singleWpts Trajectory Control DEBUG only/Pre-traitement ==
  In1 : Inport
  Enable : EnablePort
  Constant : Constant  Value=0
  Display : Display
  Matrix Concatenate : Concatenate  Mode=Multidimensional array
  Selector : Selector  NumberOfDimensions=2  InputPortWidth=3  IndexOptions=Index vector (dialog),Index vector (dialog)  Indices=[1:3],[1:2]  OutputSizes=1,1
  Selector1 : Selector  NumberOfDimensions=2  InputPortWidth=3  IndexOptions=Index vector (dialog),Index vector (dialog)  Indices=[4:7],[1:2]  OutputSizes=1,1
  Selector2 : Selector  NumberOfDimensions=2  InputPortWidth=3  IndexOptions=Index vector (dialog),Index vector (dialog)  Indices=[8],[2]  OutputSizes=1,1
  Selector3 : Selector  NumberOfDimensions=2  InputPortWidth=3  IndexOptions=Index vector (dialog),Index vector (dialog)  Indices=[9],[2]  OutputSizes=1,1
  Selector4 : Selector  NumberOfDimensions=2  InputPortWidth=3  IndexOptions=Index vector (dialog),Index vector (dialog)  Indices=[1:7],[2]  OutputSizes=1,1
  Terminator : Terminator
  Transpose : Math  Operator=transpose
  linWpts : Outport
  RotWpts : Outport  Port=2
  time : Outport  Port=3
  target : Outport  Port=4
  wires:
  In1/1 -> Transpose/1
  Transpose/1 -> Display/1, Selector4/1, Selector3/1, Selector2/1, Selector1/1, Selector/1
  Selector/1 -> linWpts/1
  Selector1/1 -> RotWpts/1
  Constant/1 -> Matrix Concatenate/1
  Selector2/1 -> Matrix Concatenate/2
  Matrix Concatenate/1 -> time/1
  Selector3/1 -> Terminator/1
  Selector4/1 -> target/1

== system proc_control_lite/Subsystem Trajectory/singleWpts Trajectory Control DEBUG only/Resettable Subsystem ==
  linWpts : Inport
  rotWpts : Inport  Port=2
  time : Inport  Port=3
  Reset : ResetPort  DisableCoverage=on
  Constant : Constant
  Discrete-Time Integrator : DiscreteIntegrator  IntegratorMethod=Integration: Trapezoidal  SampleTime=-1  ICPrevOutput=DiscIntNeverNeededParam  ICPrevScaledInput=DiscIntNeverNeededParam
  Rotation Trajectory : robotcorelib/Rotation Trajectory  WaypointFormat=Quaternion  WaypointSource=External  R0=[ 1, 0, 0, 0 ]'  RF=[ 0, 0, 1, 0 ]'  TimeInterval=[ 0, 1 ]  CustomTimeScaling=off  ParameterSource=Internal  TSTime=0:0.1:1  TimeScaling=[ 0:0.1:1; ones( 1, 11 ); zeros( 1, 11 ) ]  SimulateUsing=Code generation
      settings: LibrarySourceBlock=robotutilslib/Rotation Trajectory
  Selector : Selector  NumberOfDimensions=2  InputPortWidth=3  IndexOptions=Index vector (dialog),Index vector (dialog)  Indices=[1:4],1  OutputSizes=1,1
  Selector1 : Selector  NumberOfDimensions=2  InputPortWidth=3  IndexOptions=Index vector (dialog),Index vector (dialog)  Indices=[1:4],1  OutputSizes=1,1
  Subsystem : Subsystem
  Terminator : Terminator
  n1 : Outport
  epsilon : Outport  Port=2
  v1 : Outport  Port=3
  v2 : Outport  Port=4
  wires:
  Rotation Trajectory/3 -> Terminator/1
  time/1 -> Subsystem/3(time), Rotation Trajectory/4
  Constant/1 -> Discrete-Time Integrator/1
  linWpts/1 -> Subsystem/2(linWpts)
  Rotation Trajectory/1 -> epsilon/1
  Selector1/1 -> Rotation Trajectory/3
  Subsystem/1(n1) -> n1/1
  rotWpts/1 -> Selector1/1, Selector/1
  Discrete-Time Integrator/1 -> Rotation Trajectory/1, Subsystem/1(In1)
  Rotation Trajectory/2 -> v2/1
  Selector/1 -> Rotation Trajectory/2
  Subsystem/2(v1) -> v1/1

== system proc_control_lite/Subsystem Trajectory/singleWpts Trajectory Control DEBUG only/Subsystem ==
  Bus Creator : BusCreator  Inputs=3
  Bus Creator1 : BusCreator  Inputs=3
  Bus Creator2 : BusCreator  Inputs=6
  Constant{1..6} (6 alike) : Constant  Value=0
  Frame : Constant
  fine : Constant
  speed : Constant
  speed1 : Constant
  Out1 : Outport
  wires:
  Constant4/1 -> Bus Creator/1  "x"
  Constant6/1 -> Bus Creator1/1  "x"
  Bus Creator1/1 -> Bus Creator2/4  "orientation"
  Constant2/1 -> Bus Creator/2  "y"
  Constant3/1 -> Bus Creator/3  "z"
  Frame/1 -> Bus Creator2/1  "frame"
  Constant1/1 -> Bus Creator1/2  "y"
  Constant5/1 -> Bus Creator1/3  "z"
  speed/1 -> Bus Creator2/2  "speed"
  Bus Creator/1 -> Bus Creator2/3  "position"
  fine/1 -> Bus Creator2/5  "fine"
  speed1/1 -> Bus Creator2/6  "rotation"
  Bus Creator2/1 -> Out1/1

== system proc_control_lite/Ros Command/Get_ROS_param/MPC Parameters/MPC Gains ==
  Bus Creator : BusCreator  Inputs=9
  Data Type Conversion : DataTypeConversion  OutDataTypeStr=double  SaturateOnIntegerOverflow=off  RndMeth=Floor
  Data Type Conversion1 : DataTypeConversion  OutDataTypeStr=double  SaturateOnIntegerOverflow=off  RndMeth=Floor
  Gains Default : Subsystem
  Gains Mode 10 : Subsystem
  Gains Mode 11 : Subsystem
  Gains Mode 19 : Subsystem
  Gains No DVL : Subsystem
  M : ros2lib/Get Parameter  ParameterName=proc_control.mpc.m  ParameterType=int64  ParameterMaxArrayLength=64  ParameterInitialValue=MPC.m  SampleTime=-1  ModelName=proc_control_lite  BlockId=ParamGet_proc_control_lite_143
  P : ros2lib/Get Parameter  ParameterName=proc_control.mpc.p  ParameterType=double  ParameterMaxArrayLength=64  ParameterInitialValue=MPC.p  SampleTime=-1  ModelName=proc_control_lite  BlockId=ParamGet_proc_control_lite_140
  T Max : ros2lib/Get Parameter  ParameterName=proc_control.mpc.tmax  ParameterType=double  ParameterMaxArrayLength=64  ParameterInitialValue=MPC.tmax  SampleTime=-1  ModelName=proc_control_lite  BlockId=ParamGet_proc_control_lite_144
  T Min : ros2lib/Get Parameter  ParameterName=proc_control.mpc.tmin  ParameterType=double  ParameterMaxArrayLength=64  ParameterInitialValue=MPC.tmin  SampleTime=-1  ModelName=proc_control_lite  BlockId=ParamGet_proc_control_lite_145
  gains : Outport
  wires:
  P/1 -> Data Type Conversion/1  "p"
  Gains Mode 11/1(c11) -> Bus Creator/3
  M/1 -> Data Type Conversion1/1  "m"
  Data Type Conversion/1 -> Bus Creator/6  "p"
  Gains Default/1(default) -> Bus Creator/1
  Gains Mode 10/1(c10) -> Bus Creator/2
  Gains No DVL/1(noDvl) -> Bus Creator/5
  Gains Mode 19/1(c19) -> Bus Creator/4
  Data Type Conversion1/1 -> Bus Creator/7  "m"
  T Max/1 -> Bus Creator/8  "tmax"
  T Min/1 -> Bus Creator/9  "tmin"
  Bus Creator/1 -> gains/1  "gains"

== system proc_control_lite/Ros Command/Get_ROS_param/MPC Parameters/targetReached Params ==
  Angular Tolerance : ros2lib/Get Parameter  ParameterName=proc_control.target_reached.angular_tolerance  ParameterType=double  ParameterMaxArrayLength=16  ParameterInitialValue=MPC.targetReached.angularTol  SampleTime=-1  ModelName=proc_control_lite  BlockId=ParamGet_proc_control_lite_151
  Bus Creator : BusCreator  Inputs=3
  Linear Tolerance : ros2lib/Get Parameter  ParameterName=proc_control.target_reached.linear_tolerance  ParameterType=double  ParameterMaxArrayLength=16  ParameterInitialValue=MPC.targetReached.linearTol  SampleTime=-1  ModelName=proc_control_lite  BlockId=ParamGet_proc_control_lite_150
  Time In Tolerance : ros2lib/Get Parameter  ParameterName=proc_control.target_reached.time_in_tolerance  ParameterType=double  ParameterMaxArrayLength=16  ParameterInitialValue=MPC.targetReached.timeInTol  SampleTime=-1  ModelName=proc_control_lite  BlockId=ParamGet_proc_control_lite_152
  targetReached : Outport
  wires:
  Linear Tolerance/1 -> Bus Creator/1  "linearTol"
  Angular Tolerance/1 -> Bus Creator/2  "angularTol"
  Time In Tolerance/1 -> Bus Creator/3  "timeInTol"
  Bus Creator/1 -> targetReached/1  "targetReached"

== system proc_control_lite/Subsystem Controller/Controller List/If Action Subsystem/Bus2Mux ==
  Mo : Inport
  Bus Selector : BusSelector  OutputSignals=WorldPosition,qS2W,Body Velocity,Angular Rate
  Mux : Mux
  n1 : Outport
  wires:
  Mo/1 -> Bus Selector/1
  Mux/1 -> n1/1
  Bus Selector/2 -> Mux/2  "<qS2W>"
  Bus Selector/1 -> Mux/1  "<WorldPosition>"
  Bus Selector/3 -> Mux/3  "<Body Velocity>"
  Bus Selector/4 -> Mux/4  "<Angular Rate>"

== system proc_control_lite/Subsystem Controller/Controller List/If Action Subsystem/Sent mesurement residuals ==
  In1 : Inport
  Blank Message : ros2lib/Blank Message  messageClass=Message  entityType=nav_msgs/Odometry  messageType=nav_msgs/Odometry  SampleTime=-1
  Bus Assignment : BusAssignment  AssignedSignals=pose.pose.position.x,pose.pose.position.y,pose.pose.position.z,pose.pose.orientation.w,pose.pose.orientation.x,pose.pose.orientation.y,pose.pose.orientation.z,twist.twist.linear.x,twist.twist.linear.y,twist.twist.linear.z,twist.twist.angular.x,twist.twist.angular.y,twist.twist.angular.z
  Demux : Demux  Outputs=13
  Header Assignment : ros2lib/Header Assignment  SetFrameID=on  FrameID=NED  InsertTimeStamp=on  SetHeaderFieldName=Use the default header field name  HeaderFieldName=header
  Publish : ros2lib/Publish  topicSource=Specify your own  topic=/proc_control/measurment_residual  messageType=nav_msgs/Odometry  QOSHistory=Keep last  QOSDepth=1  QOSReliability=Reliable  QOSDurability=Volatile  QOSDeadline=Inf  QOSLifespan=Inf  QOSLiveliness=Automatic  QOSLeaseDuration=Inf  QOSAvoidROSNamespaceConventions=off
  wires:
  Blank Message/1 -> Header Assignment/1
  Header Assignment/1 -> Bus Assignment/1
  Demux/1 -> Bus Assignment/2
  Demux/2 -> Bus Assignment/3
  Demux/3 -> Bus Assignment/4
  Demux/4 -> Bus Assignment/6
  Demux/5 -> Bus Assignment/5
  Demux/6 -> Bus Assignment/7
  Demux/7 -> Bus Assignment/8
  Demux/8 -> Bus Assignment/9
  Demux/9 -> Bus Assignment/10
  Demux/10 -> Bus Assignment/11
  Demux/11 -> Bus Assignment/12
  Demux/12 -> Bus Assignment/13
  Demux/13 -> Bus Assignment/14
  In1/1 -> Demux/1
  Bus Assignment/1 -> Publish/1

== system proc_control_lite/Subsystem Controller/Controller List/If Action Subsystem1/Bus2Mux ==
  Mo : Inport
  Bus Selector : BusSelector  OutputSignals=WorldPosition,qS2W,Body Velocity,Angular Rate
  Mux : Mux
  Out1 : Outport
  wires:
  Mo/1 -> Bus Selector/1
  Bus Selector/1 -> Mux/1  "<WorldPosition>"
  Bus Selector/2 -> Mux/2  "<qS2W>"
  Bus Selector/3 -> Mux/3  "<Body Velocity>"
  Bus Selector/4 -> Mux/4  "<Angular Rate>"
  Mux/1 -> Out1/1

== system proc_control_lite/Subsystem Controller/Controller List/Quaternion Non linear MPC (Not for codegen)/Bus2Mux1 ==
  Mo : Inport
  Bus Selector : BusSelector  OutputSignals=WorldPosition,qS2W,Body Velocity,Angular Rate
  Mux : Mux
  Out1 : Outport
  wires:
  Mo/1 -> Bus Selector/1
  Bus Selector/1 -> Mux/1  "<WorldPosition>"
  Bus Selector/2 -> Mux/2  "<qS2W>"
  Bus Selector/3 -> Mux/3  "<Body Velocity>"
  Bus Selector/4 -> Mux/4  "<Angular Rate>"
  Mux/1 -> Out1/1

== system proc_control_lite/Subsystem Controller/If Action Subsystem/Subsystem/Subsystem ==
  Bus Creator : BusCreator  Inputs=2
  Constant : Constant  Value=uint32(0)
  Constant1 : Constant  Value=uint32(0)
  Out1 : Outport
  wires:
  Constant/1 -> Bus Creator/1  "CurrentLength"
  Bus Creator/1 -> Out1/1
  Constant1/1 -> Bus Creator/2  "ReceivedLength"

== system proc_control_lite/Subsystem Controller/If Action Subsystem/Subsystem/Subsystem1 ==
  Bus Creator : BusCreator  Inputs=2
  Constant : Constant  Value=uint32(0)
  Constant1 : Constant  Value=uint32(0)
  Out1 : Outport
  wires:
  Bus Creator/1 -> Out1/1
  Constant/1 -> Bus Creator/1  "CurrentLength"
  Constant1/1 -> Bus Creator/2  "ReceivedLength"

== system proc_control_lite/Subsystem Controller/If Action Subsystem/Subsystem/Subsystem2 ==
  Bus Creator : BusCreator  Inputs=2
  Constant : Constant  Value=uint32(0)
  Constant1 : Constant  Value=uint32(0)
  Out1 : Outport
  wires:
  Bus Creator/1 -> Out1/1
  Constant/1 -> Bus Creator/1  "CurrentLength"
  Constant1/1 -> Bus Creator/2  "ReceivedLength"
